simulink model "PID"  (R2022a)
settings: Solver=VariableStepAuto  StartTime=0.0  StopTime=1000.0  RelTol=1e-3
settings Model: Creator=HHQ  LastModifiedBy=HHQ

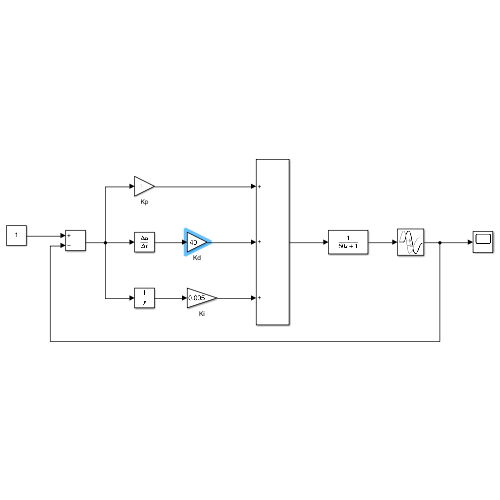
[thumbnail: Simulink's stored preview of the top-level diagram]
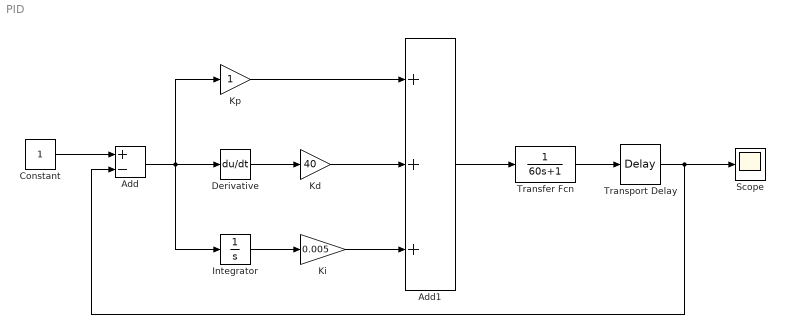
== system PID ==
  Add : Sum  Inputs=+-
  Add1 : Sum  Inputs=+++
  Constant : Constant
  Derivative : Derivative
  Integrator : Integrator
  Kd : Gain  Gain=40
  Ki : Gain  Gain=0.005
  Kp : Gain
  Scope : Scope
  Transfer Fcn : TransferFcn  Denominator=[60 1]
  Transport Delay : TransportDelay  DelayTime=80
  wires:
  Constant/1 -> Add/1
  Add/1 -> Integrator/1, Derivative/1, Kp/1
  Integrator/1 -> Ki/1
  Derivative/1 -> Kd/1
  Kp/1 -> Add1/1
  Add1/1 -> Transfer Fcn/1
  Transfer Fcn/1 -> Transport Delay/1
  Transport Delay/1 -> Add/2, Scope/1
  Ki/1 -> Add1/3
  Kd/1 -> Add1/2
